simulink model "sim_polytrajD5"  (R2020b)
settings: Solver=VariableStepAuto  StartTime=0.0  StopTime=10.0  RelTol=1e-3
settings Model: Creator=mstra  LastModifiedBy=mstra

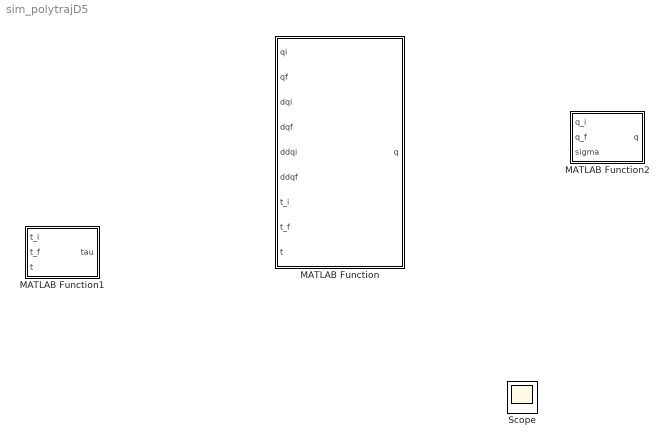
== system sim_polytrajD5 ==
  MATLAB Function : MATLAB Function  TreatAsAtomicUnit=on
  MATLAB Function1 : MATLAB Function  TreatAsAtomicUnit=on
  MATLAB Function2 : MATLAB Function  TreatAsAtomicUnit=on
  Scope : Scope

== matlab function sim_polytrajD5/MATLAB Function1 ==
  data: t_i input; tau output; t_f input; t input
function tau = t2tau(t_i,t_f,t)
%Change parameter to tau

T = t_f - t_i;
tau = (t - t_i)/T;

== matlab function sim_polytrajD5/MATLAB Function ==
  data: qi input; qf input; q output; dqi input; dqf input; ddqi input; ddqf input; t_i input; t_f input; t input
function q  = sim_poly_trajD5(qi, qf ,dqi ,dqf ,ddqi ,ddqf, t_i, t_f, t)
%make quintic polynomial

v = [qi dqi ddqi qf dqf ddqf]';

A = [1 t_i t_i^2 t_i^3 t_i^4 t_i^5; 
     0 1 2*t_i 3*t_i^2 4*t_i^3 5*t_i^4; 
     0 0 2 6*t_i 12*t_i^2 20*t_i^3; 
     1 t_f t_f^2 t_f^3 t_f^4 t_f^5;
     0 1 2*t_f 3*t_f^2 4*t_f^3 5*t_f^4;
     0 0 2 6*t_f 12*t_f^2 20*t_f^3];
 
% invert to get the coefficients
a = inv(A)*v;

% trying the matrix way
q = a(1,1) + a(2,1)*(t-t_i) + a(3,1)*(t-t_i)^2 + a(4,1)*(t-t_i)^3 + a(5,1)*(t-t_i)^4 + a(6,1)*(t-t_i)^5;
% return position at t

end

== matlab function sim_polytrajD5/MATLAB Function2 ==
  data: q_i input; q output; q_f input; sigma input
function q = fcn(q_i,q_f,sigma)
%parameter normalisation

h = q_f - q_i;
q = q_i + h * sigma;
